simulink model "ControlAdapter"  (R2023a)
settings: Solver=VariableStepAuto  StartTime=0.0  StopTime=10.0  RelTol=1e-3
settings Model: Creator=romav  LastModifiedBy=romav

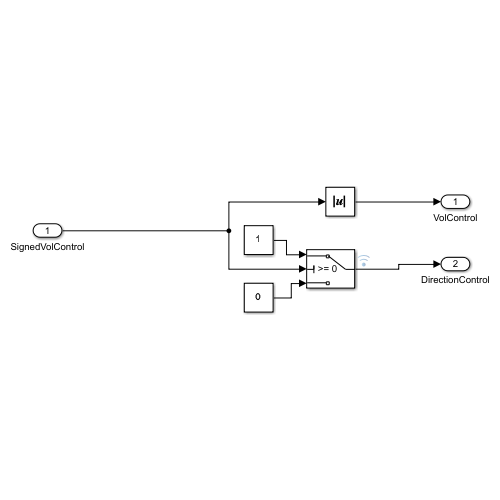
[thumbnail: Simulink's stored preview of the top-level diagram]
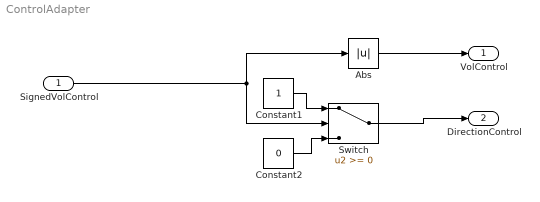
== system ControlAdapter ==
  SignedVolControl : Inport
  Abs : Abs  SaturateOnIntegerOverflow=off
  Constant1 : Constant
  Constant2 : Constant  Value=0
  Switch : Switch  ZeroCross=off  SaturateOnIntegerOverflow=off  InputSameDT=off
  VolControl : Outport
  DirectionControl : Outport  Port=2
  wires:
  Abs/1 -> VolControl/1
  Constant1/1 -> Switch/1
  SignedVolControl/1 -> Abs/1, Switch/2
  Constant2/1 -> Switch/3
  Switch/1 -> DirectionControl/1
